simulink model "R7014E_DoubleTankSim"  (R2018a)
settings: Solver=ode5  StartTime=0.0  StopTime=500  RelTol=1e-3  EnableMultiTasking=on
Description:
  | Double tank process simulation model
  | V1.0
  | 
  | Author: Wolfgang Birk, LTU
settings Model: MinMaxOverflowLogging=ForceOff  Creator=wolfgang  LastModifiedBy=anttib-5
settings DataIOCC: LimitDataPoints=on  SaveFormat=Array  SignalLoggingSaveFormat=ModelDataLogs
settings OptimizationCC: ExpressionDepthLimit=2147483647  LifeSpan=inf
settings DebuggingCC: UnderspecifiedInitializationDetection=Classic  MergeDetectMultiDrivingBlocksExec=none  SolverPrmCheckMsg=warning  FcnCallInpInsideContextMsg=warning  StateNameClashWarn=warning  SFUnexpectedBacktrackingDiag=warning  SFNoUnconditionalDefaultTransitionDiag=warning  SFExecutionAtInitializationDiag=none
settings HardwareCC: ProdBitPerPointer=32  ProdBitPerSizeT=32  ProdBitPerPtrDiffT=32  ProdLargestAtomicFloat=None  ProdIntDivRoundTo=Undefined  ProdEndianess=Unspecified  ProdWordSize=32  ProdHWDeviceType=32-bit Generic
settings ModelReferenceCC: PropagateSignalLabelsOutOfModel=off
settings CodeAppCC: StateflowObjectComments=on
settings GRTTargetCC: TargetLangStandard=C89/C90 (ANSI)  GeneratePreprocessorConditionals=Disable all
settings ConfigComp: CovMetricSettings=dw  CovHtmlReporting=on  CovSaveCumulativeToWorkspaceVar=on  CovSaveSingleToWorkspaceVar=on  CovExternalEMLEnable=off

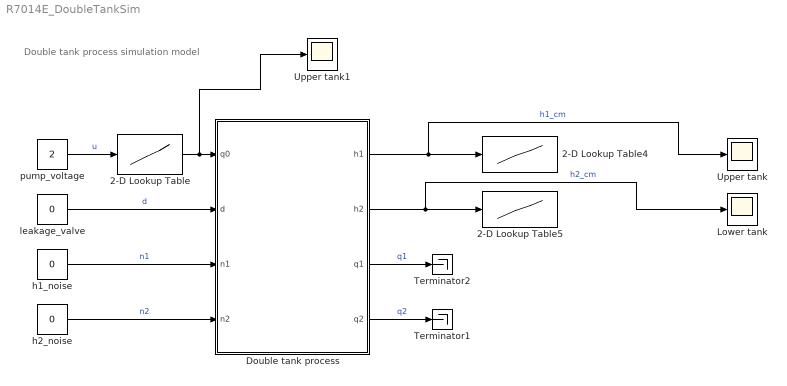
== system R7014E_DoubleTankSim ==
  note: Double tank process simulation model
  2-D Lookup Table : Lookup_n-D  NumberOfTableDimensions=1  BreakpointsForDimension1=x  BreakpointsForDimension2=[1:3]  Table=y  RndMeth=Simplest  InputSameDT=on  mask{x=[0,1,2,3,4,5,6,7,8,9,10], y=[0, 18.86, 28.53, 34.42, 38.82, 42.86, 45.47,47.87, 51, 52, 53.95]}
      mask prompts: x "Values on x-axis"; y "Values on y-axis"
  2-D Lookup Table4 : Lookup_n-D  NumberOfTableDimensions=1  BreakpointsForDimension1=x  BreakpointsForDimension2=[1:3]  Table=y  RndMeth=Simplest  InputSameDT=on  mask{x=[0, 3.4, 5, 6.8, 8.4, 9.7, 11, 12, 13, 14.2, 15.1], y=[0, 0.90, 2.17, 3.54, 4.79, 5.9, 6.997, 7.78, 8.53, 9.395, 9.995]}
      mask prompts: x "Values on x-axis"; y "Values on y-axis"
  2-D Lookup Table5 : Lookup_n-D  NumberOfTableDimensions=1  BreakpointsForDimension1=x  BreakpointsForDimension2=[1:3]  Table=y  RndMeth=Simplest  InputSameDT=on  mask{x=[0, 4.4, 5, 6.1, 7.3, 8.5, 9.6, 10.6, 12, 13.2, 14.7], y=[0, 1.04, 1.71, 2.32, 3.19, 4.11, 5.03, 5.77, 6.68, 7.64, 8.69]}
      mask prompts: x "Values on x-axis"; y "Values on y-axis"
  Double tank process : Subsystem  mask{At=33, Ao=0.17, hmax=15.5}
      mask prompts: At "Tank area (cm^2)"; Ao "Opening area (cm^2)"; hmax "Tank height (cm)"
      mask help: Double tank process parameters
  Lower tank : Scope
  Terminator1 : Terminator
  Terminator2 : Terminator
  Upper tank : Scope
  Upper tank1 : Scope
  h1_noise : Constant  Value=0
  h2_noise : Constant  Value=0
  leakage_valve : Constant  Value=0
  pump_voltage : Constant  Value=2
  wires:
  leakage_valve/1 -> Double tank process/2(d)  "d"
  pump_voltage/1 -> 2-D Lookup Table/1  "u"
  Double tank process/1(h1) -> 2-D Lookup Table4/1, Upper tank/1  "h1_cm"
  Double tank process/2(h2) -> 2-D Lookup Table5/1, Lower tank/1  "h2_cm"
  Double tank process/4(q2) -> Terminator1/1  "q2"
  Double tank process/3(q1) -> Terminator2/1  "q1"
  h1_noise/1 -> Double tank process/3(n1)  "n1"
  h2_noise/1 -> Double tank process/4(n2)  "n2"
  2-D Lookup Table/1 -> Upper tank1/1, Double tank process/1(q0)

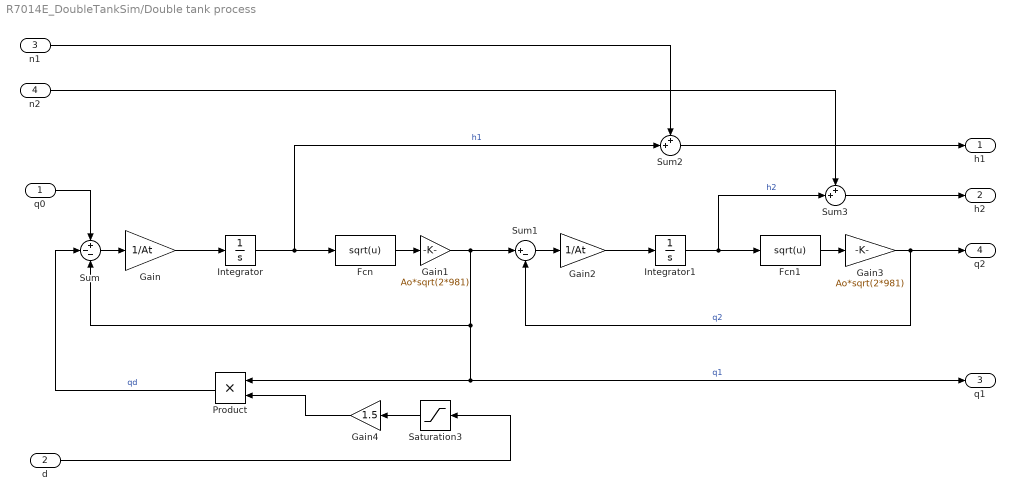
== system R7014E_DoubleTankSim/Double tank process ==
  q0 : Inport
  d : Inport  Port=2
  n1 : Inport  Port=3
  n2 : Inport  Port=4
  Fcn : Fcn  Expr=sqrt(u)
  Fcn1 : Fcn  Expr=sqrt(u)
  Gain : Gain  Gain=1/At
  Gain1 : Gain  Gain=Ao*sqrt(2*981)
  Gain2 : Gain  Gain=1/At
  Gain3 : Gain  Gain=Ao*sqrt(2*981)
  Gain4 : Gain  Gain=1.5
  Integrator : Integrator  LimitOutput=on  UpperSaturationLimit=hmax  LowerSaturationLimit=0
  Integrator1 : Integrator  LimitOutput=on  UpperSaturationLimit=hmax  LowerSaturationLimit=0
  Product : Product  RndMeth=Zero
  Saturation3 : Saturate  UpperLimit=1  LowerLimit=0
  Sum : Sum  Inputs=+--
  Sum1 : Sum  Inputs=|+-
  Sum2 : Sum  Inputs=++|
  Sum3 : Sum  Inputs=++|
  h1 : Outport
  h2 : Outport  Port=2
  q1 : Outport  Port=3
  q2 : Outport  Port=4
  wires:
  Sum/1 -> Gain/1
  Gain/1 -> Integrator/1
  Fcn/1 -> Gain1/1
  Gain1/1 -> Sum1/1, Product/1, q1/1, Sum/3  "q1"
  Sum1/1 -> Gain2/1
  Gain2/1 -> Integrator1/1
  Fcn1/1 -> Gain3/1
  Gain3/1 -> Sum1/2, q2/1  "q2"
  q0/1 -> Sum/1
  Integrator/1 -> Sum2/2, Fcn/1  "h1"
  Product/1 -> Sum/2  "qd"
  d/1 -> Saturation3/1
  Integrator1/1 -> Sum3/2, Fcn1/1  "h2"
  Saturation3/1 -> Gain4/1
  Gain4/1 -> Product/2
  Sum2/1 -> h1/1
  n1/1 -> Sum2/1
  Sum3/1 -> h2/1
  n2/1 -> Sum3/1
